simulink model "PlantnMPC"  (R2020b)
settings: Solver=VariableStepAuto  StartTime=0.0  StopTime=100  RelTol=1e-3
undefined symbols (not defined in the file): dU0, magnitude, U0
settings Model: Creator=firda  LastModifiedBy=firda

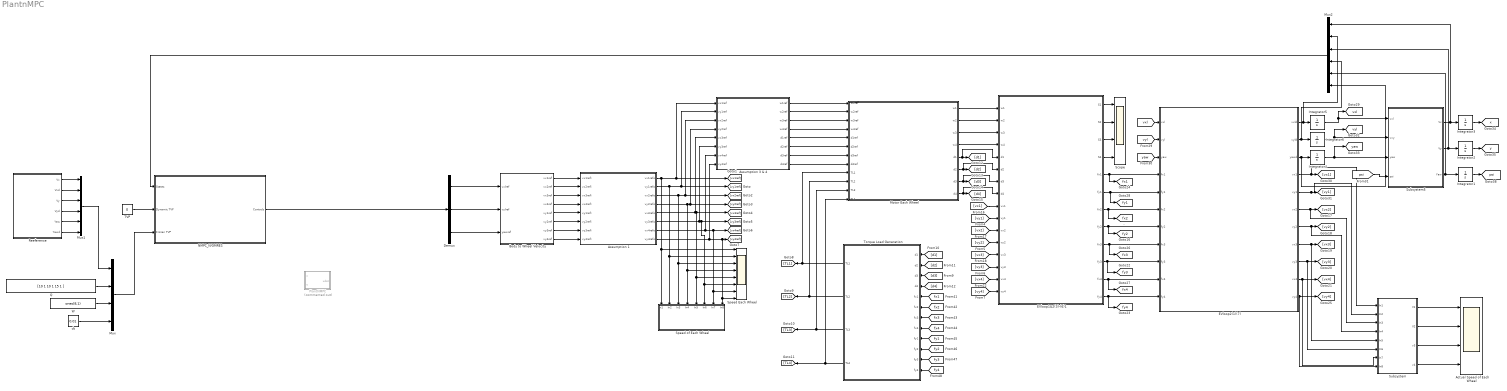
== system PlantnMPC ==
  Actual Speed of Each Wheel : Scope  NumInputPorts=4
  Assumption 1 : Subsystem  mask(Ketentuan ICM){}
      mask help:
      | djref tidak terdefinisi ketika vxjref=vyjref=0
      | vxjref dan vyjref mengambil nilai sebelumnya saat keduanya sama dengan nol
  Assumption 3 & 4 : Subsystem  mask(Persamaan ICM){rej=0.32}
      mask prompts: rej "Jari-jari roda (m)"
      mask help:
      | Asumsi 3 (Zero Slip), bidang roda berhimpit dengan Vj, aj=0,
      | djref=sudut apit (vxjref dan vyjref)
      | Asumsi 4 (Free Rolling), slip longitudinal SLj=0,
      | wjref= norm(vxjref,vyjref)/rej
  Body to Wheel Velocity : Subsystem  mask(Persamaan ICM){ld=0.75, lf=1.42, lr=1.42}
      mask prompts: ld "Jarak pusat masa ke bodi samping (m)"; lf "Jarak pusat masa ke bodi depan (m)"; lr "Jarak pusat masa ke bodi belakang (m)"
      mask help:
      | mengkoordinasikan kecepatan masing-masing roda
      | terhadap kecepatan pusat kendaraan
      | dengan menggunakan konsep ICM
  Demux : Demux  Outputs=3
  EVloop1&2(3)-(6)1 : Subsystem  mask(Vehicle body dinamic){re1=0.32, re2=0.32, re3=0.32, re4=0.32, m=1000, g=9.8, h=0.42, ld=0.75, lf=1.42, lr=1.42, kro=20972, kfo=50539, ksj=0.95}
      mask prompts: re1 "jari-jari roda 1 (m)"; re2 "jari-jari roda 2 (m)"; re3 "jari-jari roda 3 (m)"; re4 "jari-jari roda 4 (m)"; m "massa kendaraan (kg)"; g "percepatan gravitasi (m/s^2)"; h "tinggi pusat massa dari permukaan jalan (m)"; ld "jarak pusat massa ke bodi samping (m)"; lf "jarak pusat massa ke bodi depan (m)"; lr "jarak pusat massa ke bodi belakang (m)"; kro "ketegangan roll belakang"; kfo "ketegangan roll depan"; ksj "faktor atenuasi"
      mask help: Persamaan (3)(4)(5)(6)
  EVloop2(1)(7) : Subsystem  mask(Vehicle bodi dinamic){m=1000, ld=0.75, lf=1.42, lr=1.42, Jz=1950}
      mask prompts: m "massa kendaraan (kg)"; ld "jarak pusat massa ke bodi samping (m)"; lf "jarak pusat massa ke bodi depan (m)"; lr "jarak pusat massa ke bodi belakang (m)"; Jz "the moment of inertia of the vehicle about an axis through its CM"
      mask help: Loop 2 Persamaan 1 & 7
  Integrator{1..4,6} (5 alike) : Integrator
  Integrator5 : Integrator  InitialCondition=1.6
  Motor Each Wheel : Subsystem
      mask Display: image('C:\Users\firda\Desktop\Scenario\4wheels.jpg'); % Use "Edit Image" on toolstrip to change.
  Mux : Mux
  Mux1 : Mux  Inputs=6
  Mux2 : Mux  Inputs=6
  NMPC_N/GMRES : Subsystem
  PlantNMPC : MATLAB Function  Commented=on  TreatAsAtomicUnit=on
  Q : Constant  Value=[10 1 10 1 15 1 ]
  Reeference : Subsystem
      mask Display: image('Reference.jpg'); % Use "Edit Image" on toolstrip to change.
  Scope : Scope  NumInputPorts=4
  Speed Each Wheel : Scope  NumInputPorts=8
  Speed of Each Wheel : Subsystem
  Subsystem : Subsystem
  Subsystem5 : Subsystem
  TVP : Constant  Value=0
  Torque Load Generation : Subsystem  mask(Vehicle body dinamic){jm1=0.36, jm2=0.36, jm3=0.36, jm4=0.36, re1=0.32, re2=0.32, re3=0.32, re4=0.32}
      mask prompts: jm1 "momen inersia roda 1 (kgm^2)"; jm2 "momen inersia roda 2 (kgm^2)"; jm3 "momen inersia roda 3 (kgm^2)"; jm4 "momen inersia roda 4 (kgm^2)"; re1 "jari-jari roda 1 (m)"; re2 "jari-jari roda 2 (m)"; re3 "jari-jari roda 3 (m)"; re4 "jari-jari roda 4 (m)"
      mask help: Persamaan (9)
  W : Constant  Value=ones(8,1)
  dt : Constant  Value=0.01
  tag scope: fx1=global, fx2=global, fx3=global, fx4=global, fy1=global, fy2=global, fy3=global, fy4=global, psi=global, vxl=global, vyl=global, x=global, y=global, yaw=global
  wires:
  Assumption 1/1(vx1refo) -> Assumption 3 & 4/1(vx1ref), [vx1ref], Speed of Each Wheel/1(In1), Speed Each Wheel/1
  Assumption 1/2(vy1refo) -> Assumption 3 & 4/2(vy1ref), [vy1ref], Speed Each Wheel/2, Speed of Each Wheel/2(In2)
  Assumption 1/3(vx2refo) -> Assumption 3 & 4/3(vx2ref), [vx2ref], Speed Each Wheel/3, Speed of Each Wheel/3(In3)
  Assumption 1/4(vy2refo) -> [vy2ref], Assumption 3 & 4/4(vy2ref), Speed of Each Wheel/4(In4), Speed Each Wheel/4
  Assumption 1/5(vx3refo) -> Speed Each Wheel/5, Speed of Each Wheel/5(In5), [vx3ref], Assumption 3 & 4/5(vx3ref)
  Assumption 1/6(vy3refo) -> [vy3ref], Speed Each Wheel/6, Speed of Each Wheel/6(In6), Assumption 3 & 4/6(vy3ref)
  Assumption 1/7(vx4refo) -> [vx4ref], Speed Each Wheel/7, Speed of Each Wheel/7(In7), Assumption 3 & 4/7(vx4ref)
  Assumption 1/8(vy4refo) -> Speed Each Wheel/8, Speed of Each Wheel/8(In8), [vy4ref], Assumption 3 & 4/8(vy4ref)
  Assumption 3 & 4/1(w1ref) -> Motor Each Wheel/1(w1ref)
  Assumption 3 & 4/2(w2ref) -> Motor Each Wheel/2(w2ref)
  Assumption 3 & 4/3(w3ref) -> Motor Each Wheel/3(w3ref)
  Assumption 3 & 4/4(w4ref) -> Motor Each Wheel/4(w4ref)
  Assumption 3 & 4/5(d1ref) -> Motor Each Wheel/5(d1ref)
  Assumption 3 & 4/6(d2ref) -> Motor Each Wheel/6(d2ref)
  Assumption 3 & 4/7(d3ref) -> Motor Each Wheel/7(d3ref)
  Assumption 3 & 4/8(d4ref) -> Motor Each Wheel/8(d4ref)
  Torque Load Generation/3(TL3) -> Motor Each Wheel/11(TL3), [TL3]
  Torque Load Generation/4(TL4) -> Motor Each Wheel/12(TL4), [TL4]
  Torque Load Generation/1(TL1) -> Motor Each Wheel/9(TL1), [TL1]
  [d1] -> Torque Load Generation/1(d1)
  [d2] -> Torque Load Generation/2(d2)
  [d3] -> Torque Load Generation/3(d3)
  [d4] -> Torque Load Generation/4(d4)
  [fx1] -> Torque Load Generation/5(fx1)
  [fx2] -> Torque Load Generation/6(fx2)
  [fx3] -> Torque Load Generation/7(fx3)
  [fx4] -> Torque Load Generation/8(fx4)
  [fy1] -> Torque Load Generation/9(fy1)
  [fy2] -> Torque Load Generation/10(fy2)
  [fy3] -> Torque Load Generation/11(fy3)
  [fy4] -> Torque Load Generation/12(fy4)
  Torque Load Generation/2(TL2) -> [TL2], Motor Each Wheel/10(TL2)
  Motor Each Wheel/1(w1) -> EVloop1&2(3)-(6)1/1(w1)
  Motor Each Wheel/2(w2) -> EVloop1&2(3)-(6)1/2(w2)
  Motor Each Wheel/3(w3) -> EVloop1&2(3)-(6)1/3(w3)
  Motor Each Wheel/4(w4) -> EVloop1&2(3)-(6)1/4(w4)
  Motor Each Wheel/6(d2) -> EVloop1&2(3)-(6)1/6(d2), [d2]
  Motor Each Wheel/7(d3) -> EVloop1&2(3)-(6)1/7(d3), [d3]
  Motor Each Wheel/8(d4) -> EVloop1&2(3)-(6)1/8(d4), [d4]
  Motor Each Wheel/5(d1) -> EVloop1&2(3)-(6)1/5(d1), [d1]
  [vx1] -> EVloop1&2(3)-(6)1/9(vx1)
  [vy1] -> EVloop1&2(3)-(6)1/10(vy1)
  [vx2] -> EVloop1&2(3)-(6)1/11(vx2)
  [vy4] -> EVloop1&2(3)-(6)1/16(vy4)
  [vx4] -> EVloop1&2(3)-(6)1/15(vx4)
  [vy3] -> EVloop1&2(3)-(6)1/14(vy3)
  [vx3] -> EVloop1&2(3)-(6)1/13(vx3)
  [vy2] -> EVloop1&2(3)-(6)1/12(vy2)
  EVloop1&2(3)-(6)1/1(S1) -> Scope/1
  EVloop1&2(3)-(6)1/2(S2) -> Scope/2
  EVloop1&2(3)-(6)1/3(S3) -> Scope/3
  EVloop1&2(3)-(6)1/4(S4) -> Scope/4
  EVloop1&2(3)-(6)1/5(fx1) -> [fx1], EVloop2(1)(7)/4(fx1)
  EVloop1&2(3)-(6)1/6(fy1) -> [fy1], EVloop2(1)(7)/5(fy1)
  EVloop1&2(3)-(6)1/7(fx2) -> [fx2], EVloop2(1)(7)/6(fx2)
  EVloop1&2(3)-(6)1/8(fy2) -> [fy2], EVloop2(1)(7)/7(fy2)
  EVloop1&2(3)-(6)1/9(fx3) -> [fx3], EVloop2(1)(7)/8(fx3)
  EVloop1&2(3)-(6)1/10(fy3) -> [fy3], EVloop2(1)(7)/9(fy3)
  EVloop1&2(3)-(6)1/11(fx4) -> [fx4], EVloop2(1)(7)/10(fx4)
  EVloop1&2(3)-(6)1/12(fy4) -> [fy4], EVloop2(1)(7)/11(fy4)
  [vxl] -> EVloop2(1)(7)/1(vxl)
  [vyl] -> EVloop2(1)(7)/2(vyl)
  [yaw] -> EVloop2(1)(7)/3(yaw)
  Integrator4/1 -> Subsystem5/3(yaw), [yaw]
  Integrator6/1 -> Subsystem5/2(vxy), [vyl]
  Integrator5/1 -> Subsystem5/1(vxl), [vxl]
  EVloop2(1)(7)/1(vxld) -> Mux2/2, Integrator5/1
  EVloop2(1)(7)/2(vyld) -> Mux2/4, Integrator6/1
  EVloop2(1)(7)/3(yawd) -> Mux2/6, Integrator4/1
  [psi] -> Subsystem5/4(psi)
  Integrator2/1 -> [y]
  Subsystem5/1(Vx) -> Mux2/1, Integrator3/1
  Integrator3/1 -> [x]
  Integrator1/1 -> [psi]
  Subsystem5/2(Vy) -> Mux2/3, Integrator2/1
  Subsystem5/3(Yaw) -> Integrator1/1, Mux2/5
  EVloop2(1)(7)/4(vx1) -> Subsystem/1(In1), [vx1]
  EVloop2(1)(7)/5(vy1) -> Subsystem/2(In2), [vy1]
  EVloop2(1)(7)/6(vx2) -> Subsystem/3(In3), [vx2]
  EVloop2(1)(7)/7(vy2) -> Subsystem/4(In4), [vy2]
  EVloop2(1)(7)/8(vx3) -> Subsystem/5(In5), [vx3]
  EVloop2(1)(7)/9(vy3) -> Subsystem/6(In6), [vy3]
  EVloop2(1)(7)/10(vx4) -> Subsystem/7(In7), [vx4]
  EVloop2(1)(7)/11(vy4) -> Subsystem/8(In8), [vy4]
  Subsystem/1(V1) -> Actual Speed of Each Wheel/1
  Subsystem/2(V2) -> Actual Speed of Each Wheel/2
  Subsystem/3(v3) -> Actual Speed of Each Wheel/3
  Subsystem/4(v4) -> Actual Speed of Each Wheel/4
  Body to Wheel Velocity/8(vy4ref) -> Assumption 1/8(vy4refi)
  Body to Wheel Velocity/7(vy3ref) -> Assumption 1/7(vy3refi)
  Body to Wheel Velocity/6(vy2ref) -> Assumption 1/6(vy2refi)
  Body to Wheel Velocity/5(vy1ref) -> Assumption 1/5(vy1refi)
  Body to Wheel Velocity/4(vx4ref) -> Assumption 1/4(vx4refi)
  Body to Wheel Velocity/3(vx3ref) -> Assumption 1/3(vx3refi)
  Body to Wheel Velocity/2(vx2ref) -> Assumption 1/2(vx2refi)
  Body to Wheel Velocity/1(vx1ref) -> Assumption 1/1(vx1refi)
  Demux/1 -> Body to Wheel Velocity/1(vxlref)
  Demux/2 -> Body to Wheel Velocity/2(vylref)
  Demux/3 -> Body to Wheel Velocity/3(yawref)
  Q/1 -> Mux/2
  dt/1 -> Mux/4
  W/1 -> Mux/3
  Mux/1 -> NMPC_N/GMRES/3(Frozen TVP)
  Mux1/1 -> Mux/1
  Reeference/1(Vx) -> Mux1/1
  Reeference/2(Vxd) -> Mux1/2
  Reeference/3(Vy) -> Mux1/3
  Reeference/4(Vyd) -> Mux1/4
  Reeference/5(Yaw) -> Mux1/5
  Reeference/6(Yawd) -> Mux1/6
  TVP/1 -> NMPC_N/GMRES/2(Dynamic TVP)
  NMPC_N/GMRES/1(Controls) -> Demux/1
  Mux2/1 -> NMPC_N/GMRES/1(States)

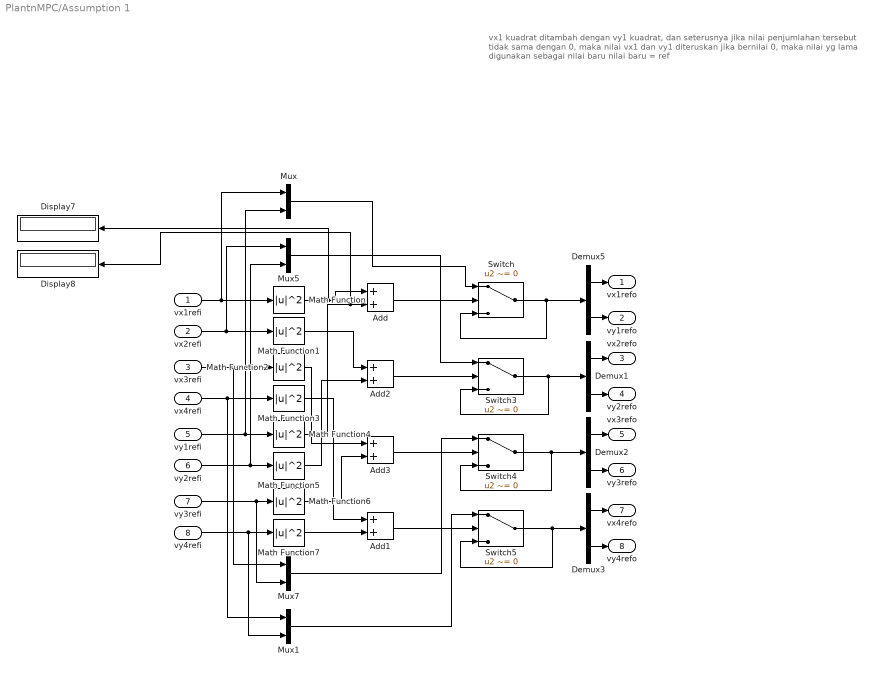
== system PlantnMPC/Assumption 1 ==
  note: vx1 kuadrat ditambah dengan vy1 kuadrat, dan seterusnya
      | jika nilai penjumlahan tersebut tidak sama dengan 0, maka nilai vx1 dan vy1 diteruskan
      | jika bernilai 0, maka nilai yg lama digunakan sebagai nilai baru
      | nilai baru = ref
  vx1refi : Inport
  vx2refi : Inport  Port=2
  vx3refi : Inport  Port=3
  vx4refi : Inport  Port=4
  vy1refi : Inport  Port=5
  vy2refi : Inport  Port=6
  vy3refi : Inport  Port=7
  vy4refi : Inport  Port=8
  Add{,1..3} (4 alike) : Sum
  Demux{1..3,5} (4 alike) : Demux  Outputs=2
  Display7 : Display
  Display8 : Display
  Math Function{,1..7} (8 alike) : Math  Operator=magnitude^2  SignedPower=on  SaturateOnIntegerOverflow=on
  Mux{,1,5,7} (4 alike) : Mux  Inputs=2
  Switch{,3..5} (4 alike) : Switch  Criteria=u2 ~= 0
  vx1refo : Outport
  vy1refo : Outport  Port=2
  vx2refo : Outport  Port=3
  vy2refo : Outport  Port=4
  vx3refo : Outport  Port=5
  vy3refo : Outport  Port=6
  vx4refo : Outport  Port=7
  vy4refo : Outport  Port=8
  wires:
  Add2/1 -> Switch3/2
  Switch3/1 -> Switch3/3, Demux1/1
  Math Function3/1 -> Add1/1
  Demux3/2 -> vy4refo/1
  Demux5/1 -> vx1refo/1
  Demux2/1 -> vx3refo/1
  Demux3/1 -> vx4refo/1
  Math Function5/1 -> Add2/2
  vx3refi/1 -> Mux7/1, Math Function2/1
  Switch4/1 -> Switch4/3, Demux2/1
  vx2refi/1 -> Math Function1/1, Mux5/1
  Math Function6/1 -> Add3/2
  vy4refi/1 -> Mux1/2, Math Function7/1
  Math Function/1 -> Display7/1, Add/1
  Mux5/1 -> Switch3/1
  Add/1 -> Switch/2
  Mux7/1 -> Switch4/1
  Add3/1 -> Switch4/2
  Switch5/1 -> Switch5/3, Demux3/1
  Math Function2/1 -> Add3/1
  vx4refi/1 -> Mux1/1, Math Function3/1
  vy3refi/1 -> Mux7/2, Math Function6/1
  vy2refi/1 -> Mux5/2, Math Function5/1
  Math Function1/1 -> Add2/1
  Switch/1 -> Switch/3, Demux5/1
  vx1refi/1 -> Mux/1, Math Function/1
  Math Function4/1 -> Display8/1, Add/2
  vy1refi/1 -> Mux/2, Math Function4/1
  Mux/1 -> Switch/1
  Math Function7/1 -> Add1/2
  Add1/1 -> Switch5/2
  Demux1/1 -> vx2refo/1
  ? -> ?
  Mux1/1 -> Switch5/1
  Demux5/2 -> vy1refo/1
  Demux2/2 -> vy3refo/1
  Demux1/2 -> vy2refo/1

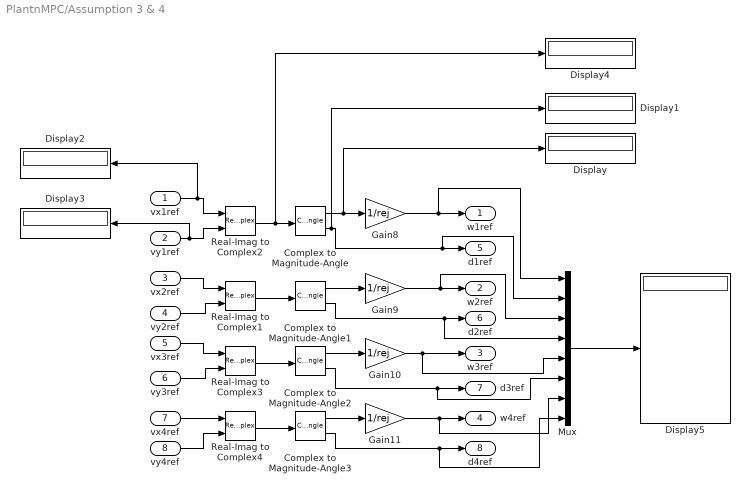
== system PlantnMPC/Assumption 3 & 4 ==
  vx1ref : Inport
  vy1ref : Inport  Port=2
  vx2ref : Inport  Port=3
  vy2ref : Inport  Port=4
  vx3ref : Inport  Port=5
  vy3ref : Inport  Port=6
  vx4ref : Inport  Port=7
  vy4ref : Inport  Port=8
  Complex to Magnitude-Angle{,1..3} (4 alike) : ComplexToMagnitudeAngle
  Display{,1..5} (6 alike) : Display
  Gain{8..11} (4 alike) : Gain  Gain=1/rej
  Mux : Mux  Inputs=8
  Real-Imag to Complex{1..4} (4 alike) : RealImagToComplex
  w1ref : Outport
  w2ref : Outport  Port=2
  w3ref : Outport  Port=3
  w4ref : Outport  Port=4
  d1ref : Outport  Port=5
  d2ref : Outport  Port=6
  d3ref : Outport  Port=7
  d4ref : Outport  Port=8
  wires:
  vx2ref/1 -> Real-Imag to Complex1/1
  vy1ref/1 -> Real-Imag to Complex2/2, Display3/1
  Gain8/1 -> Mux/1, w1ref/1
  Complex to Magnitude-Angle/2 -> Display1/1, Mux/2, d1ref/1
  Gain9/1 -> Mux/3, w2ref/1
  vy2ref/1 -> Real-Imag to Complex1/2
  Complex to Magnitude-Angle2/2 -> Mux/6, d3ref/1
  vx3ref/1 -> Real-Imag to Complex3/1
  vy4ref/1 -> Real-Imag to Complex4/2
  Complex to Magnitude-Angle3/1 -> Gain11/1
  Complex to Magnitude-Angle3/2 -> Mux/8, d4ref/1
  Real-Imag to Complex1/1 -> Complex to Magnitude-Angle1/1
  Complex to Magnitude-Angle1/2 -> Mux/4, d2ref/1
  vy3ref/1 -> Real-Imag to Complex3/2
  Complex to Magnitude-Angle/1 -> Display/1, Gain8/1
  Gain11/1 -> Mux/7, w4ref/1
  vx1ref/1 -> Display2/1, Real-Imag to Complex2/1
  vx4ref/1 -> Real-Imag to Complex4/1
  Real-Imag to Complex2/1 -> Display4/1, Complex to Magnitude-Angle/1
  Complex to Magnitude-Angle1/1 -> Gain9/1
  Real-Imag to Complex3/1 -> Complex to Magnitude-Angle2/1
  Complex to Magnitude-Angle2/1 -> Gain10/1
  Real-Imag to Complex4/1 -> Complex to Magnitude-Angle3/1
  Gain10/1 -> w3ref/1, Mux/5
  Mux/1 -> Display5/1

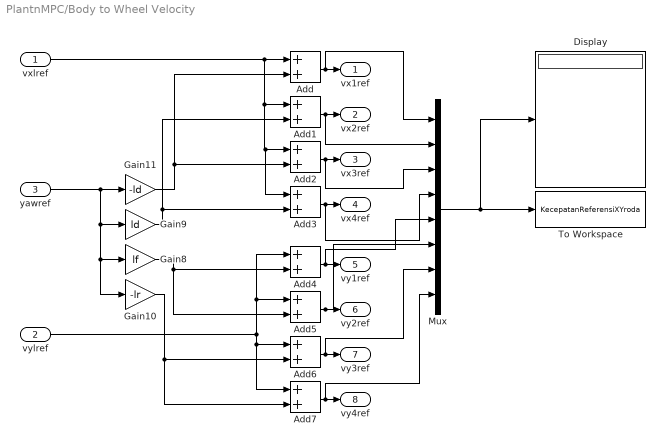
== system PlantnMPC/Body to Wheel Velocity ==
  vxlref : Inport
  vylref : Inport  Port=2
  yawref : Inport  Port=3
  Add{,1..7} (8 alike) : Sum
  Display : Display
  Gain10 : Gain  Gain=-lr
  Gain11 : Gain  Gain=-ld
  Gain8 : Gain  Gain=lf
  Gain9 : Gain  Gain=ld
  Mux : Mux  Inputs=8
  To Workspace : ToWorkspace  VariableName=KecepatanReferensiXYroda  SaveFormat=Structure With Time  SampleTime=0.01
  vx1ref : Outport
  vx2ref : Outport  Port=2
  vx3ref : Outport  Port=3
  vx4ref : Outport  Port=4
  vy1ref : Outport  Port=5
  vy2ref : Outport  Port=6
  vy3ref : Outport  Port=7
  vy4ref : Outport  Port=8
  wires:
  Gain10/1 -> Add7/2, Add6/2
  Add1/1 -> Mux/2, vx2ref/1
  Gain8/1 -> Add4/2, Add5/2
  yawref/1 -> Gain9/1, Gain8/1, Gain10/1, Gain11/1
  vylref/1 -> Add7/1, Add6/1, Add5/1, Add4/1
  vxlref/1 -> Add3/1, Add2/1, Add1/1, Add/1
  Gain9/1 -> Add1/2, Add3/2
  Gain11/1 -> Add2/2, Add/2
  Add3/1 -> Mux/4, vx4ref/1
  Add/1 -> Mux/1, vx1ref/1
  Add5/1 -> Mux/6, vy2ref/1
  Add2/1 -> Mux/3, vx3ref/1
  Add4/1 -> Mux/5, vy1ref/1
  Add6/1 -> Mux/7, vy3ref/1
  Add7/1 -> Mux/8, vy4ref/1
  Mux/1 -> Display/1, To Workspace/1

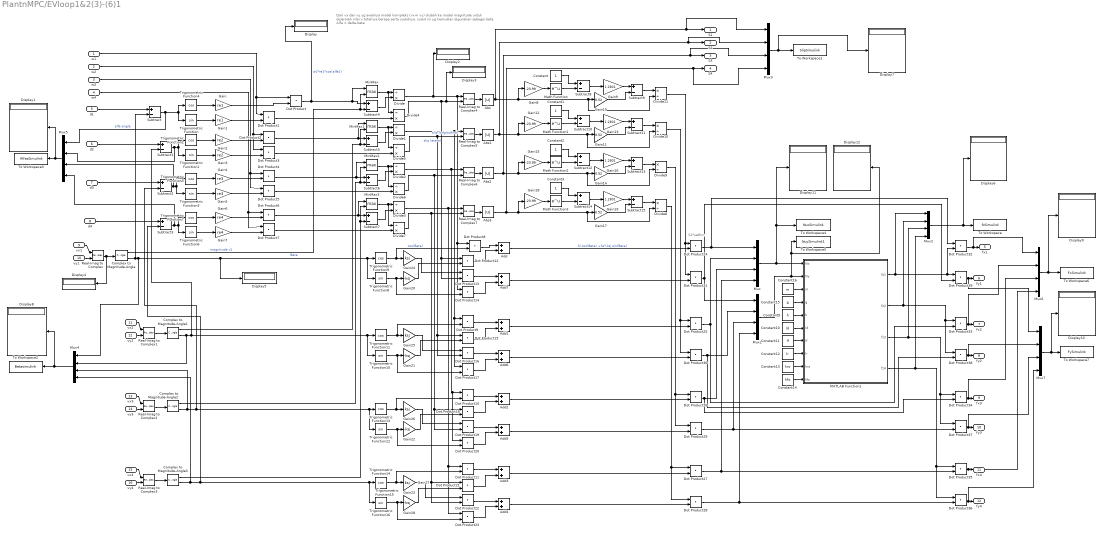
== system PlantnMPC/EVloop1&2(3)-(6)1 ==
  note: S1*satfcn
  note: Dari vx dan vy yg awalnya model kompleks (vx+i vy) diubah ke model magnitude untuk diperoleh nilai v totalnya berapa serta sudutnya. sudut ini yg kemudian digunakan sebagai beta.
      | Alfa = delta-beta
  w1 : Inport
  w2 : Inport  Port=2
  w3 : Inport  Port=3
  w4 : Inport  Port=4
  d1 : Inport  Port=5
  d2 : Inport  Port=6
  d3 : Inport  Port=7
  d4 : Inport  Port=8
  vx1 : Inport  Port=9
  vy1 : Inport  Port=10
  vx2 : Inport  Port=11
  vy2 : Inport  Port=12
  vx3 : Inport  Port=13
  vy3 : Inport  Port=14
  vx4 : Inport  Port=15
  vy4 : Inport  Port=16
  Abs{,1..3} (4 alike) : Abs
  Add{,1..7} (8 alike) : Sum
  Complex to Magnitude-Angle{,1..3} (4 alike) : ComplexToMagnitudeAngle
  Constant{,1..3} (4 alike) : Constant
  Constant10 : Constant  Value=ld
  Constant11 : Constant  Value=lf
  Constant12 : Constant  Value=lr
  Constant13 : Constant  Value=kro
  Constant14 : Constant  Value=kfo
  Constant15 : Constant  Value=g
  Constant16 : Constant  Value=m
  Constant9 : Constant  Value=h
  Display{,1..12} (13 alike) : Display
  Divide{,1..7} (8 alike) : Product  Inputs=/*
  Divide{8..11} (4 alike) : Product  Inputs=*/
  Dot Product{,1..39} (40 alike) : DotProduct  InputSameDT=on  OutDataTypeStr=Inherit: Inherit via internal rule
  Gain : Gain  Gain=re1
  Gain1 : Gain  Gain=re1
  Gain{10..11,14,17} (4 alike) : Gain  Gain=0.52
  Gain{8,12,15,18} (4 alike) : Gain  Gain=-23.99
  Gain{9,13,16,19} (4 alike) : Gain  Gain=1.2801
  Gain2 : Gain  Gain=re2
  Gain{20..23,28} (5 alike) : Gain  Gain=-ksj
  Gain{24..27} (4 alike) : Gain  Gain=ksj
  Gain3 : Gain  Gain=re2
  Gain4 : Gain  Gain=re3
  Gain5 : Gain  Gain=re3
  Gain6 : Gain  Gain=re4
  Gain7 : Gain  Gain=re4
  MATLAB Function1 : MATLAB Function  TreatAsAtomicUnit=on
  Math Function{,1..3} (4 alike) : Math  SignedPower=on  SaturateOnIntegerOverflow=on
  MinMax{,1..3} (4 alike) : MinMax  Function=max  Inputs=2
  Mux{,1..7} (8 alike) : Mux
  Real-Imag to Complex{,1..7} (8 alike) : RealImagToComplex
  Subtract{,1..15} (16 alike) : Sum  Inputs=+-
  To Workspace : ToWorkspace  VariableName=fzSimulink  SaveFormat=Structure With Time  SampleTime=0.01
      settings: Save2DSignal=2-D array (concatenate along first dimension)
  To Workspace1 : ToWorkspace  VariableName=SlipSimulink  SaveFormat=Structure With Time  SampleTime=0.01
  To Workspace2 : ToWorkspace  VariableName=Betasimulink  SaveFormat=Structure With Time  SampleTime=0.01
  To Workspace3 : ToWorkspace  VariableName=AlfasSimulink  SaveFormat=Structure With Time  SampleTime=0.01
  To Workspace4 : ToWorkspace  VariableName=NuxSimulink  SaveFormat=Structure With Time  SampleTime=0.01
  To Workspace5 : ToWorkspace  VariableName=NuySimulink1  SaveFormat=Structure With Time  SampleTime=0.01
  To Workspace6 : ToWorkspace  VariableName=FxSimulink  SaveFormat=Structure With Time  SampleTime=0.01
  To Workspace7 : ToWorkspace  VariableName=FySimulink  SaveFormat=Structure With Time  SampleTime=0.01
  Trigonometric Function{,1,3,6,8,10,12,14,16} (9 alike) : Trigonometry
  Trigonometric Function{2,4..5,7,9,11,13,15} (8 alike) : Trigonometry  Operator=cos
  S1 : Outport
  S2 : Outport  Port=2
  S3 : Outport  Port=3
  S4 : Outport  Port=4
  fx1 : Outport  Port=5
  fy1 : Outport  Port=6
  fx2 : Outport  Port=7
  fy2 : Outport  Port=8
  fx3 : Outport  Port=9
  fy3 : Outport  Port=10
  fx4 : Outport  Port=11
  fy4 : Outport  Port=12
  wires:
  Dot Product33/1 -> Mux6/2, fx2/1
  Dot Product35/1 -> Mux6/4, fx4/1
  Dot Product28/1 -> Dot Product36/2, Mux1/4
  Dot Product36/1 -> Mux7/4, fy4/1
  Dot Product34/1 -> Mux6/3, fx3/1
  Dot Product39/1 -> Mux7/1, fy1/1
  Dot Product37/1 -> Mux7/3, fy3/1
  Dot Product38/1 -> Mux7/2, fy2/1
  Dot Product32/1 -> Mux6/1, fx1/1
  vx1/1 -> Real-Imag to Complex/1
  vy1/1 -> Real-Imag to Complex/2
  vx3/1 -> Real-Imag to Complex2/1
  vy3/1 -> Real-Imag to Complex2/2
  vx4/1 -> Real-Imag to Complex3/1
  vx2/1 -> Real-Imag to Complex1/1
  vy4/1 -> Real-Imag to Complex3/2
  vy2/1 -> Real-Imag to Complex1/2
  Constant15/1 -> MATLAB Function1/4(g)
  Dot Product31/1 -> Dot Product39/2, Mux1/1
  Dot Product29/1 -> Dot Product37/2, Mux1/3
  Dot Product30/1 -> Dot Product38/2, Mux1/2
  Constant16/1 -> MATLAB Function1/3(m)
  MATLAB Function1/1(fz1) -> Mux2/1, Dot Product32/2, Dot Product39/1
  MATLAB Function1/3(fz3) -> Mux2/3, Dot Product34/1, Dot Product37/1
  Constant14/1 -> MATLAB Function1/10(kfo)
  Constant13/1 -> MATLAB Function1/9(kro)
  Real-Imag to Complex2/1 -> Complex to Magnitude-Angle2/1
  Real-Imag to Complex3/1 -> Complex to Magnitude-Angle3/1
  Complex to Magnitude-Angle/2 -> Mux4/1, Display5/1, Trigonometric Function8/1, Trigonometric Function9/1, Subtract/2  "Beta"
  Complex to Magnitude-Angle1/2 -> Mux4/2, Trigonometric Function10/1, Trigonometric Function11/1, Subtract1/2
  Real-Imag to Complex/1 -> Display4/1, Complex to Magnitude-Angle/1
  Real-Imag to Complex1/1 -> Complex to Magnitude-Angle1/1
  Trigonometric Function1/1 -> Gain3/1
  w1/1 -> Dot Product1/1, Dot Product/1
  Trigonometric Function5/1 -> Gain4/1
  d4/1 -> Subtract3/1
  Subtract/1 -> Mux5/1, Trigonometric Function/1, Trigonometric Function4/1  "alfa angle"
  Gain4/1 -> Dot Product4/2
  w2/1 -> Dot Product2/1, Dot Product3/1
  w4/1 -> Dot Product6/1, Dot Product7/1
  Subtract2/1 -> Mux5/3, Trigonometric Function3/1, Trigonometric Function5/1
  d3/1 -> Subtract2/1
  Gain5/1 -> Dot Product5/2
  Gain/1 -> Dot Product/2
  Dot Product2/1 -> MinMax1/1, Subtract5/1
  Gain1/1 -> Dot Product1/2
  d1/1 -> Subtract/1
  Gain3/1 -> Dot Product3/2
  Gain7/1 -> Dot Product7/2
  Trigonometric Function6/1 -> Gain7/1
  Dot Product/1 -> Display/1, Subtract4/1, MinMax/1  "w1*re1*cos(alfa1)"
  Complex to Magnitude-Angle3/2 -> Mux4/4, Subtract3/2, Trigonometric Function16/1, Trigonometric Function14/1, Trigonometric Function15/1
  Trigonometric Function4/1 -> Gain/1
  Complex to Magnitude-Angle2/2 -> Mux4/3, Trigonometric Function12/1, Trigonometric Function13/1, Subtract2/2
  Subtract1/1 -> Mux5/2, Trigonometric Function2/1, Trigonometric Function1/1
  Trigonometric Function2/1 -> Gain2/1
  Trigonometric Function3/1 -> Gain5/1
  Gain6/1 -> Dot Product6/2
  Trigonometric Function/1 -> Gain1/1
  Gain2/1 -> Dot Product2/2
  w3/1 -> Dot Product4/1, Dot Product5/1
  Trigonometric Function7/1 -> Gain6/1
  d2/1 -> Subtract1/1
  Subtract3/1 -> Mux5/4, Trigonometric Function6/1, Trigonometric Function7/1
  Complex to Magnitude-Angle/1 -> MinMax/2, Subtract4/2  "magnitude v1"
  Real-Imag to Complex5/1 -> Abs1/1
  Divide3/1 -> Dot Product23/1, Dot Product11/1, Real-Imag to Complex7/1
  Dot Product5/1 -> Divide6/2
  Divide/1 -> Display2/1, Dot Product14/1, Dot Product8/1, Real-Imag to Complex4/1  "slip longitudinal"
  Real-Imag to Complex6/1 -> Abs2/1
  MinMax3/1 -> Divide7/1, Divide3/1
  Divide7/1 -> Dot Product22/2, Dot Product21/1, Real-Imag to Complex7/2
  MinMax1/1 -> Divide5/1, Divide1/1
  Dot Product3/1 -> Divide5/2
  Dot Product7/1 -> Divide7/2
  Subtract5/1 -> Divide1/2
  Divide6/1 -> Dot Product19/2, Dot Product18/1, Real-Imag to Complex6/2
  Real-Imag to Complex7/1 -> Abs3/1
  Complex to Magnitude-Angle3/1 -> MinMax3/2, Subtract7/2
  Dot Product4/1 -> MinMax2/1, Subtract6/1
  Dot Product6/1 -> MinMax3/1, Subtract7/1
  Real-Imag to Complex4/1 -> Abs/1
  Gain8/1 -> Math Function/1
  Subtract6/1 -> Divide2/2
  Math Function/1 -> Subtract8/2
  Divide4/1 -> Dot Product13/2, Dot Product12/1, Display3/1, Real-Imag to Complex4/2  "slip lateral"
  Complex to Magnitude-Angle2/1 -> MinMax2/2, Subtract6/2
  Dot Product1/1 -> Divide4/2
  Subtract4/1 -> Divide/2
  Complex to Magnitude-Angle1/1 -> MinMax1/2, Subtract5/2
  MinMax/1 -> Divide4/1, Divide/1
  Subtract7/1 -> Divide3/2
  Divide5/1 -> Dot Product15/1, Dot Product16/2, Real-Imag to Complex5/2
  Divide2/1 -> Dot Product20/1, Dot Product10/1, Real-Imag to Complex6/1
  MinMax2/1 -> Divide6/1, Divide2/1
  Divide1/1 -> Dot Product9/1, Dot Product17/1, Real-Imag to Complex5/1
  Gain9/1 -> Subtract9/1
  Gain12/1 -> Math Function1/1
  Trigonometric Function8/1 -> Dot Product14/2, Gain20/1
  Trigonometric Function10/1 -> Dot Product17/2, Gain21/1
  Gain10/1 -> Subtract9/2
  Subtract8/1 -> Gain9/1
  Trigonometric Function14/1 -> Gain23/1
  Subtract14/1 -> Gain19/1
  Abs3/1 -> Mux3/4, S4/1, Gain18/1, Gain17/1, Divide8/2
  Abs2/1 -> Mux3/3, S3/1, Gain15/1, Divide9/2, Gain14/1
  Subtract13/1 -> Divide9/1
  Subtract10/1 -> Gain13/1
  Gain18/1 -> Math Function3/1
  Subtract15/1 -> Divide8/1
  Constant2/1 -> Subtract12/1
  Constant1/1 -> Subtract10/1
  Constant3/1 -> Subtract14/1
  Trigonometric Function12/1 -> Dot Product20/2, Gain22/1
  Abs1/1 -> Mux3/2, S2/1, Gain12/1, Divide10/2, Gain11/1
  Trigonometric Function9/1 -> Dot Product8/2, Gain24/1  "cos(Beta)"
  Gain16/1 -> Subtract13/1
  Gain17/1 -> Subtract15/2
  Constant/1 -> Subtract8/1
  Math Function1/1 -> Subtract10/2
  Gain13/1 -> Subtract11/1
  Math Function2/1 -> Subtract12/2
  Subtract12/1 -> Gain16/1
  Gain15/1 -> Math Function2/1
  Gain14/1 -> Subtract13/2
  Math Function3/1 -> Subtract14/2
  Gain19/1 -> Subtract15/1
  Gain11/1 -> Subtract11/2
  Divide9/1 -> Dot Product26/1, Dot Product29/1
  Dot Product11/1 -> Add3/1
  Trigonometric Function13/1 -> Dot Product10/2, Gain26/1
  Add3/1 -> Dot Product27/2
  Dot Product10/1 -> Add2/1
  Add2/1 -> Dot Product26/2
  Dot Product21/1 -> Add3/2
  Divide8/1 -> Dot Product28/1, Dot Product27/1
  Trigonometric Function16/1 -> Dot Product23/2, Gain28/1
  Gain24/1 -> Dot Product13/1
  Dot Product9/1 -> Add1/1
  Gain25/1 -> Dot Product16/1
  Gain26/1 -> Dot Product19/1
  Add4/1 -> Dot Product28/2
  Divide11/1 -> Dot Product31/1, Dot Product24/1
  Dot Product18/1 -> Add2/2
  Add/1 -> Dot Product24/2  "Sl cos(Beta) +Ss*-ksj sin(Beta)"
  Gain20/1 -> Dot Product12/2
  Dot Product8/1 -> Add/1
  Gain21/1 -> Dot Product15/2
  Gain22/1 -> Dot Product18/2
  Dot Product15/1 -> Add1/2
  Divide10/1 -> Dot Product30/1, Dot Product25/1
  Abs/1 -> Mux3/1, S1/1, Gain8/1, Divide11/2, Gain10/1
  Trigonometric Function11/1 -> Dot Product9/2, Gain25/1
  Gain28/1 -> Dot Product21/2
  Trigonometric Function15/1 -> Dot Product11/2, Gain27/1
  Subtract9/1 -> Divide11/1
  Add1/1 -> Dot Product25/2
  Dot Product12/1 -> Add/2
  Subtract11/1 -> Divide10/1
  Add7/1 -> Dot Product31/2
  Dot Product22/1 -> Add4/1
  Dot Product16/1 -> Add6/1
  Add5/1 -> Dot Product29/2
  Dot Product17/1 -> Add6/2
  Dot Product13/1 -> Add7/1
  Dot Product19/1 -> Add5/1
  Dot Product14/1 -> Add7/2
  Add6/1 -> Dot Product30/2
  Dot Product23/1 -> Add4/2
  Dot Product20/1 -> Add5/2
  Dot Product27/1 -> Dot Product35/2, Mux/4
  Constant11/1 -> MATLAB Function1/7(lf)
  Dot Product25/1 -> Dot Product33/2, Mux/2
  Constant9/1 -> MATLAB Function1/5(h)
  Dot Product24/1 -> Dot Product32/1, Mux/1
  Constant10/1 -> MATLAB Function1/6(ld)
  Mux1/1 -> To Workspace5/1, Display12/1, MATLAB Function1/2(Ny)
  Constant12/1 -> MATLAB Function1/8(lr)
  MATLAB Function1/4(fz4) -> Mux2/4, Dot Product36/1, Dot Product35/1
  MATLAB Function1/2(fz2) -> Mux2/2, Dot Product33/1, Dot Product38/1
  Dot Product26/1 -> Dot Product34/2, Mux/3
  Mux/1 -> Display11/1, To Workspace4/1, MATLAB Function1/1(Nx)
  Mux2/1 -> Display6/1, To Workspace/1
  Mux5/1 -> Display1/1, To Workspace3/1
  Mux3/1 -> Display7/1, To Workspace1/1
  Mux6/1 -> Display9/1, To Workspace6/1
  Mux7/1 -> Display10/1, To Workspace7/1
  Mux4/1 -> Display8/1, To Workspace2/1
  Gain27/1 -> Dot Product22/1

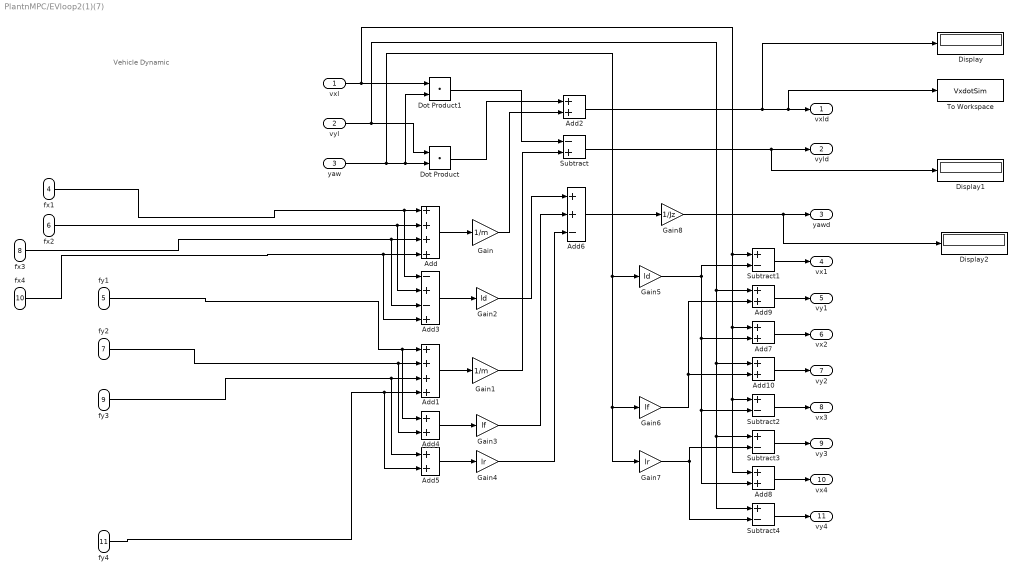
== system PlantnMPC/EVloop2(1)(7) ==
  note: Vehicle Dynamic
  vxl : Inport
  vyl : Inport  Port=2
  yaw : Inport  Port=3
  fx1 : Inport  Port=4
  fy1 : Inport  Port=5
  fx2 : Inport  Port=6
  fy2 : Inport  Port=7
  fx3 : Inport  Port=8
  fy3 : Inport  Port=9
  fx4 : Inport  Port=10
  fy4 : Inport  Port=11
  Add : Sum  Inputs=++++
  Add1 : Sum  Inputs=++++
  Add{2,4..5,7..10} (7 alike) : Sum
  Add3 : Sum  Inputs=-+-+
  Add6 : Sum  Inputs=++-
  Display : Display
  Display1 : Display
  Display2 : Display
  Dot Product : DotProduct  InputSameDT=on  OutDataTypeStr=Inherit: Inherit via internal rule
  Dot Product1 : DotProduct  InputSameDT=on  OutDataTypeStr=Inherit: Inherit via internal rule
  Gain : Gain  Gain=1/m
  Gain1 : Gain  Gain=1/m
  Gain2 : Gain  Gain=ld
  Gain3 : Gain  Gain=lf
  Gain4 : Gain  Gain=lr
  Gain5 : Gain  Gain=ld
  Gain6 : Gain  Gain=lf
  Gain7 : Gain  Gain=lr
  Gain8 : Gain  Gain=1/Jz
  Subtract : Sum  Inputs=-+
  Subtract{1..4} (4 alike) : Sum  Inputs=+-
  To Workspace : ToWorkspace  VariableName=VxdotSim  SaveFormat=Structure With Time  SampleTime=0.01
  vxld : Outport
  vyld : Outport  Port=2
  yawd : Outport  Port=3
  vx1 : Outport  Port=4
  vy1 : Outport  Port=5
  vx2 : Outport  Port=6
  vy2 : Outport  Port=7
  vx3 : Outport  Port=8
  vy3 : Outport  Port=9
  vx4 : Outport  Port=10
  vy4 : Outport  Port=11
  wires:
  Subtract3/1 -> vy3/1
  Add3/1 -> Gain2/1
  Add1/1 -> Gain1/1
  vxl/1 -> Add7/1, Subtract2/1, Add8/1, Subtract1/1, Dot Product1/1
  yaw/1 -> Gain7/1, Gain6/1, Gain5/1, Dot Product1/2, Dot Product/2
  Add8/1 -> vx4/1
  Add/1 -> Gain/1
  Gain6/1 -> Add10/2, Add9/2
  Gain1/1 -> Subtract/2
  vyl/1 -> Dot Product/1, Subtract4/1, Subtract3/1, Add10/1, Add9/1
  Add9/1 -> vy1/1
  Gain2/1 -> Add6/1
  Add4/1 -> Gain3/1
  Subtract4/1 -> vy4/1
  Subtract1/1 -> vx1/1
  Add6/1 -> Gain8/1
  Add10/1 -> vy2/1
  Dot Product/1 -> Add2/1
  Gain7/1 -> Subtract4/2, Subtract3/2
  Gain5/1 -> Add8/2, Subtract2/2, Add7/2, Subtract1/2
  Subtract2/1 -> vx3/1
  Subtract/1 -> Display1/1, vyld/1
  Dot Product1/1 -> Subtract/1
  Add7/1 -> vx2/1
  Add5/1 -> Gain4/1
  Gain3/1 -> Add6/2
  Add2/1 -> Display/1, To Workspace/1, vxld/1
  Gain/1 -> Add2/2
  fy4/1 -> Add5/2, Add1/4
  fy2/1 -> Add4/2, Add1/2
  fy3/1 -> Add5/1, Add1/3
  fy1/1 -> Add1/1, Add4/1
  fx4/1 -> Add3/4, Add/4
  fx2/1 -> Add3/2, Add/2
  fx3/1 -> Add3/3, Add/3
  fx1/1 -> Add3/1, Add/1
  Gain4/1 -> Add6/3
  Gain8/1 -> Display2/1, yawd/1

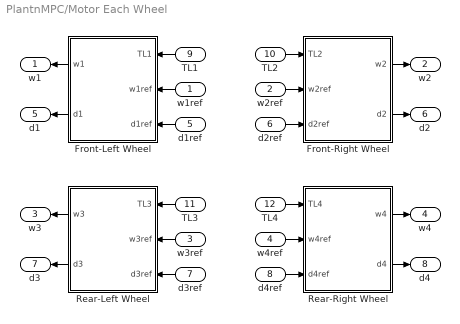
== system PlantnMPC/Motor Each Wheel ==
  w1ref : Inport
  w2ref : Inport  Port=2
  w3ref : Inport  Port=3
  w4ref : Inport  Port=4
  d1ref : Inport  Port=5
  d2ref : Inport  Port=6
  d3ref : Inport  Port=7
  d4ref : Inport  Port=8
  TL1 : Inport  Port=9
  TL2 : Inport  Port=10
  TL3 : Inport  Port=11
  TL4 : Inport  Port=12
  Front-Left Wheel : Subsystem
  Front-Right Wheel : Subsystem
  Rear-Left Wheel : Subsystem
  Rear-Right Wheel : Subsystem
  w1 : Outport
  w2 : Outport  Port=2
  w3 : Outport  Port=3
  w4 : Outport  Port=4
  d1 : Outport  Port=5
  d2 : Outport  Port=6
  d3 : Outport  Port=7
  d4 : Outport  Port=8
  wires:
  TL1/1 -> Front-Left Wheel/1(TL1)
  w1ref/1 -> Front-Left Wheel/2(w1ref)
  w2ref/1 -> Front-Right Wheel/2(w2ref)
  Front-Left Wheel/1(w1) -> w1/1
  Front-Right Wheel/1(w2) -> w2/1
  d1ref/1 -> Front-Left Wheel/3(d1ref)
  w4ref/1 -> Rear-Right Wheel/2(w4ref)
  d2ref/1 -> Front-Right Wheel/3(d2ref)
  Front-Right Wheel/2(d2) -> d2/1
  Front-Left Wheel/2(d1) -> d1/1
  Rear-Right Wheel/1(w4) -> w4/1
  Rear-Left Wheel/1(w3) -> w3/1
  w3ref/1 -> Rear-Left Wheel/2(w3ref)
  d3ref/1 -> Rear-Left Wheel/3(d3ref)
  TL2/1 -> Front-Right Wheel/1(TL2)
  TL3/1 -> Rear-Left Wheel/1(TL3)
  Rear-Left Wheel/2(d3) -> d3/1
  d4ref/1 -> Rear-Right Wheel/3(d4ref)
  TL4/1 -> Rear-Right Wheel/1(TL4)
  Rear-Right Wheel/2(d4) -> d4/1

== system PlantnMPC/NMPC_N//GMRES ==
  States : Inport
  Dynamic TVP : Inport  Port=2
  Frozen TVP : Inport  Port=3
  Solver : MATLAB Function  TreatAsAtomicUnit=on
  U0 : UnitDelay  InitialCondition=U0  SampleTime=-1  HasFrameUpgradeWarning=on
  dU0 : UnitDelay  InitialCondition=dU0  SampleTime=-1  HasFrameUpgradeWarning=on
  Controls : Outport
  wires:
  Dynamic TVP/1 -> Solver/4(TVP)
  dU0/1 -> Solver/1(dU0)
  Solver/1(dU) -> dU0/1
  U0/1 -> Solver/2(U0)
  Solver/2(U) -> U0/1
  Solver/3(Control) -> Controls/1
  Frozen TVP/1 -> Solver/5(TVP_f)
  States/1 -> Solver/3(x0)

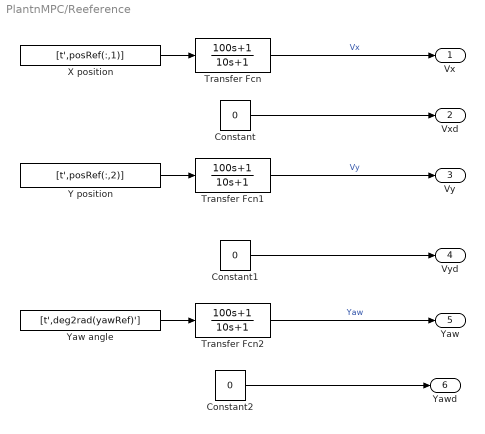
== system PlantnMPC/Reeference ==
  Constant : Constant  Value=0
  Constant1 : Constant  Value=0
  Constant2 : Constant  Value=0
  Transfer Fcn : TransferFcn  Numerator=[100 1]  Denominator=[10 1]
  Transfer Fcn1 : TransferFcn  Numerator=[100 1]  Denominator=[10 1]
  Transfer Fcn2 : TransferFcn  Numerator=[100 1]  Denominator=[10 1]
  X position : FromWorkspace  VariableName=[t',posRef(:,1)]
  Y position : FromWorkspace  VariableName=[t',posRef(:,2)]
  Yaw angle : FromWorkspace  VariableName=[t',deg2rad(yawRef)']
  Vx : Outport
  Vxd : Outport  Port=2
  Vy : Outport  Port=3
  Vyd : Outport  Port=4
  Yaw : Outport  Port=5
  Yawd : Outport  Port=6
  wires:
  X position/1 -> Transfer Fcn/1
  Yaw angle/1 -> Transfer Fcn2/1
  Y position/1 -> Transfer Fcn1/1
  Transfer Fcn1/1 -> Vy/1  "Vy"
  Transfer Fcn/1 -> Vx/1  "Vx"
  Transfer Fcn2/1 -> Yaw/1  "Yaw"
  Constant/1 -> Vxd/1
  Constant1/1 -> Vyd/1
  Constant2/1 -> Yawd/1

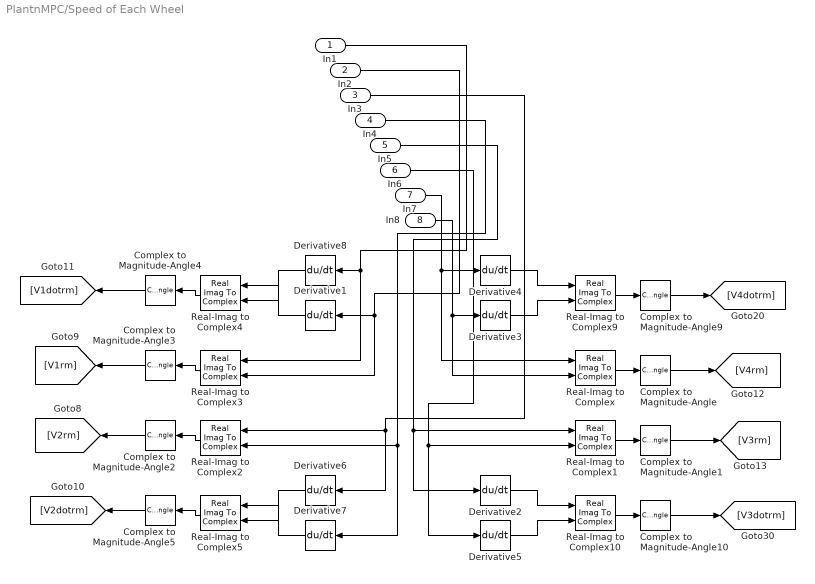
== system PlantnMPC/Speed of Each Wheel ==
  In1 : Inport
  In2 : Inport  Port=2
  In3 : Inport  Port=3
  In4 : Inport  Port=4
  In5 : Inport  Port=5
  In6 : Inport  Port=6
  In7 : Inport  Port=7
  In8 : Inport  Port=8
  Complex to Magnitude-Angle{,1..5,9..10} (8 alike) : ComplexToMagnitudeAngle  Output=Magnitude
  Derivative{1..8} (8 alike) : Derivative
  Real-Imag to Complex{,1..5,9..10} (8 alike) : RealImagToComplex
  wires:
  In2/1 -> Real-Imag to Complex3/2, Derivative1/1
  Complex to Magnitude-Angle2/1 -> [V2rm]
  In8/1 -> Real-Imag to Complex/2, Derivative3/1
  Real-Imag to Complex9/1 -> Complex to Magnitude-Angle9/1
  Real-Imag to Complex/1 -> Complex to Magnitude-Angle/1
  In3/1 -> Derivative6/1, Real-Imag to Complex2/1
  Complex to Magnitude-Angle5/1 -> [V2dotrm]
  In1/1 -> Real-Imag to Complex3/1, Derivative8/1
  Derivative7/1 -> Real-Imag to Complex5/1
  Real-Imag to Complex1/1 -> Complex to Magnitude-Angle1/1
  Real-Imag to Complex3/1 -> Complex to Magnitude-Angle3/1
  Complex to Magnitude-Angle1/1 -> [V3rm]
  In4/1 -> Derivative7/1, Real-Imag to Complex2/2
  Complex to Magnitude-Angle4/1 -> [V1dotrm]
  In6/1 -> Derivative5/1, Real-Imag to Complex1/2
  Complex to Magnitude-Angle3/1 -> [V1rm]
  Derivative8/1 -> Real-Imag to Complex4/2
  Real-Imag to Complex10/1 -> Complex to Magnitude-Angle10/1
  Derivative2/1 -> Real-Imag to Complex10/1
  Complex to Magnitude-Angle10/1 -> [V3dotrm]
  In7/1 -> Real-Imag to Complex/1, Derivative4/1
  Derivative3/1 -> Real-Imag to Complex9/2
  Complex to Magnitude-Angle9/1 -> [V4dotrm]
  In5/1 -> Derivative2/1, Real-Imag to Complex1/1
  Complex to Magnitude-Angle/1 -> [V4rm]
  Derivative4/1 -> Real-Imag to Complex9/1
  Derivative5/1 -> Real-Imag to Complex10/2
  Real-Imag to Complex5/1 -> Complex to Magnitude-Angle5/1
  Real-Imag to Complex2/1 -> Complex to Magnitude-Angle2/1
  Derivative1/1 -> Real-Imag to Complex4/1
  Derivative6/1 -> Real-Imag to Complex5/2
  Real-Imag to Complex4/1 -> Complex to Magnitude-Angle4/1

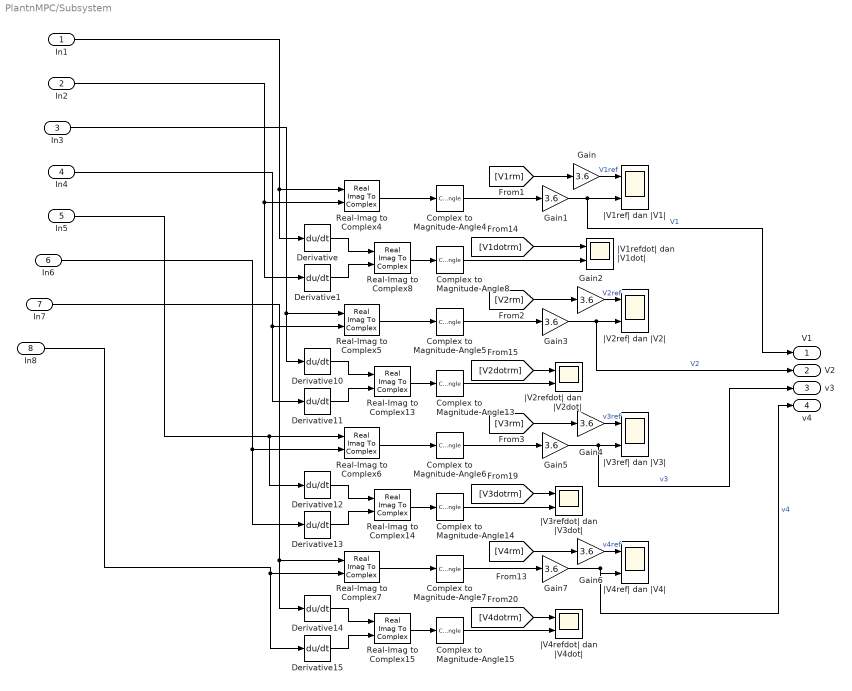
== system PlantnMPC/Subsystem ==
  In1 : Inport
  In2 : Inport  Port=2
  In3 : Inport  Port=3
  In4 : Inport  Port=4
  In5 : Inport  Port=5
  In6 : Inport  Port=6
  In7 : Inport  Port=7
  In8 : Inport  Port=8
  Complex to Magnitude-Angle{4..8,13..15} (8 alike) : ComplexToMagnitudeAngle  Output=Magnitude
  Derivative{,1,10..15} (8 alike) : Derivative
  Gain{,1..7} (8 alike) : Gain  Gain=3.6
  Real-Imag to Complex{4..8,13..15} (8 alike) : RealImagToComplex
  |V1refdot| dan |V1dot| : Scope  NumInputPorts=2
  |V1ref| dan |V1| : Scope  NumInputPorts=2
  |V2refdot| dan |V2dot| : Scope  NumInputPorts=2
  |V2ref| dan |V2| : Scope  NumInputPorts=2
  |V3refdot| dan |V3dot| : Scope  NumInputPorts=2
  |V3ref| dan |V3| : Scope  NumInputPorts=2
  |V4refdot| dan |V4dot| : Scope  NumInputPorts=2
  |V4ref| dan |V4| : Scope  NumInputPorts=2
  V1 : Outport
  V2 : Outport  Port=2
  v3 : Outport  Port=3
  v4 : Outport  Port=4
  wires:
  Real-Imag to Complex7/1 -> Complex to Magnitude-Angle7/1
  In8/1 -> Derivative15/1, Real-Imag to Complex7/2
  Derivative13/1 -> Real-Imag to Complex14/2
  In6/1 -> Derivative13/1, Real-Imag to Complex6/2
  Real-Imag to Complex15/1 -> Complex to Magnitude-Angle15/1
  Real-Imag to Complex13/1 -> Complex to Magnitude-Angle13/1
  Gain3/1 -> V2/1, |V2ref| dan |V2|/2  "V2"
  Gain2/1 -> |V2ref| dan |V2|/1  "V2ref"
  Derivative1/1 -> Real-Imag to Complex8/2
  Complex to Magnitude-Angle6/1 -> Gain5/1
  In1/1 -> Derivative/1, Real-Imag to Complex4/1
  Gain5/1 -> v3/1, |V3ref| dan |V3|/2  "v3"
  Gain7/1 -> v4/1, |V4ref| dan |V4|/2  "v4"
  In4/1 -> Derivative11/1, Real-Imag to Complex5/2
  [V4dotrm] -> |V4refdot| dan |V4dot|/1
  [V1rm] -> Gain/1
  Derivative14/1 -> Real-Imag to Complex15/1
  Derivative10/1 -> Real-Imag to Complex13/1
  Derivative12/1 -> Real-Imag to Complex14/1
  Real-Imag to Complex8/1 -> Complex to Magnitude-Angle8/1
  In5/1 -> Derivative12/1, Real-Imag to Complex6/1
  Real-Imag to Complex4/1 -> Complex to Magnitude-Angle4/1
  Gain/1 -> |V1ref| dan |V1|/1  "V1ref"
  Complex to Magnitude-Angle13/1 -> |V2refdot| dan |V2dot|/2
  Real-Imag to Complex14/1 -> Complex to Magnitude-Angle14/1
  Complex to Magnitude-Angle7/1 -> Gain7/1
  Complex to Magnitude-Angle5/1 -> Gain3/1
  Derivative/1 -> Real-Imag to Complex8/1
  [V4rm] -> Gain6/1
  [V2dotrm] -> |V2refdot| dan |V2dot|/1
  Complex to Magnitude-Angle15/1 -> |V4refdot| dan |V4dot|/2
  In2/1 -> Derivative1/1, Real-Imag to Complex4/2
  Complex to Magnitude-Angle4/1 -> Gain1/1
  [V3dotrm] -> |V3refdot| dan |V3dot|/1
  [V1dotrm] -> |V1refdot| dan |V1dot|/1
  Gain1/1 -> |V1ref| dan |V1|/2, V1/1  "V1"
  Real-Imag to Complex6/1 -> Complex to Magnitude-Angle6/1
  Real-Imag to Complex5/1 -> Complex to Magnitude-Angle5/1
  Complex to Magnitude-Angle8/1 -> |V1refdot| dan |V1dot|/2
  [V3rm] -> Gain4/1
  [V2rm] -> Gain2/1
  Gain6/1 -> |V4ref| dan |V4|/1  "v4ref"
  Gain4/1 -> |V3ref| dan |V3|/1  "v3ref"
  Derivative11/1 -> Real-Imag to Complex13/2
  Complex to Magnitude-Angle14/1 -> |V3refdot| dan |V3dot|/2
  Derivative15/1 -> Real-Imag to Complex15/2
  In3/1 -> Derivative10/1, Real-Imag to Complex5/1
  In7/1 -> Derivative14/1, Real-Imag to Complex7/1

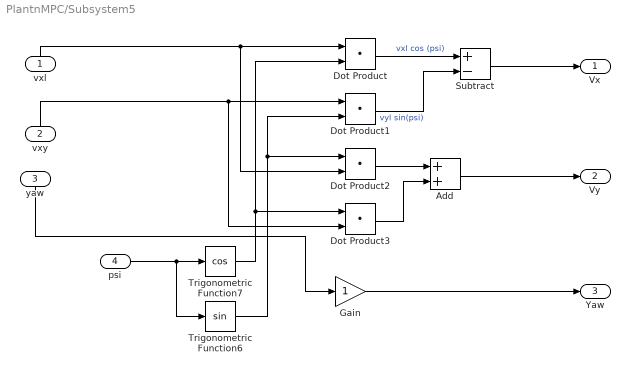
== system PlantnMPC/Subsystem5 ==
  vxl : Inport
  vxy : Inport  Port=2
  yaw : Inport  Port=3
  psi : Inport  Port=4
  Add : Sum
  Dot Product{,1..3} (4 alike) : DotProduct  InputSameDT=on  OutDataTypeStr=Inherit: Inherit via internal rule
  Gain : Gain
  Subtract : Sum  Inputs=+-
  Trigonometric Function6 : Trigonometry
  Trigonometric Function7 : Trigonometry  Operator=cos
  Vx : Outport
  Vy : Outport  Port=2
  Yaw : Outport  Port=3
  wires:
  Gain/1 -> Yaw/1
  Dot Product1/1 -> Subtract/2  "vyl sin(psi)"
  Subtract/1 -> Vx/1
  Dot Product2/1 -> Add/1
  yaw/1 -> Gain/1
  vxl/1 -> Dot Product2/2, Dot Product/1
  vxy/1 -> Dot Product3/2, Dot Product1/1
  Dot Product3/1 -> Add/2
  psi/1 -> Trigonometric Function6/1, Trigonometric Function7/1
  Trigonometric Function7/1 -> Dot Product3/1, Dot Product/2
  Trigonometric Function6/1 -> Dot Product2/1, Dot Product1/2
  Add/1 -> Vy/1
  Dot Product/1 -> Subtract/1  "vxl cos (psi)"

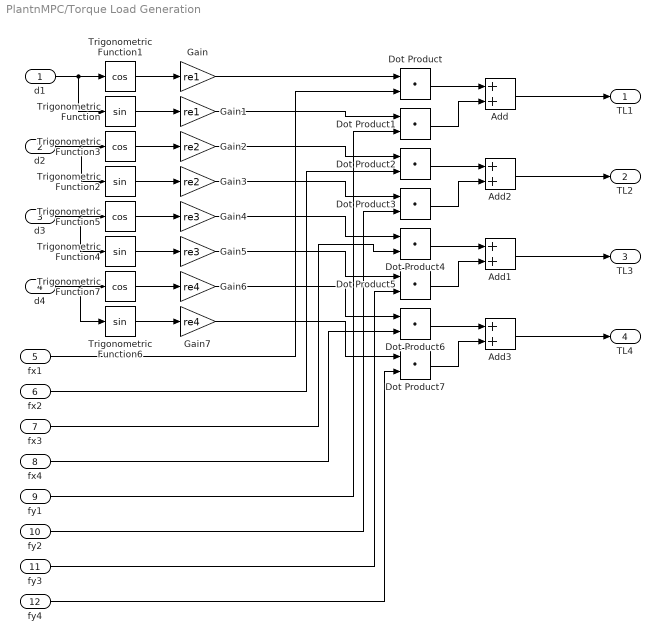
== system PlantnMPC/Torque Load Generation ==
  d1 : Inport
  d2 : Inport  Port=2
  d3 : Inport  Port=3
  d4 : Inport  Port=4
  fx1 : Inport  Port=5
  fx2 : Inport  Port=6
  fx3 : Inport  Port=7
  fx4 : Inport  Port=8
  fy1 : Inport  Port=9
  fy2 : Inport  Port=10
  fy3 : Inport  Port=11
  fy4 : Inport  Port=12
  Add{,1..3} (4 alike) : Sum
  Dot Product{,1..7} (8 alike) : DotProduct  InputSameDT=on  OutDataTypeStr=Inherit: Inherit via internal rule
  Gain : Gain  Gain=re1
  Gain1 : Gain  Gain=re1
  Gain2 : Gain  Gain=re2
  Gain3 : Gain  Gain=re2
  Gain4 : Gain  Gain=re3
  Gain5 : Gain  Gain=re3
  Gain6 : Gain  Gain=re4
  Gain7 : Gain  Gain=re4
  Trigonometric Function{,2,4,6} (4 alike) : Trigonometry
  Trigonometric Function{1,3,5,7} (4 alike) : Trigonometry  Operator=cos
  TL1 : Outport
  TL2 : Outport  Port=2
  TL3 : Outport  Port=3
  TL4 : Outport  Port=4
  wires:
  Gain3/1 -> Dot Product3/1
  fy2/1 -> Dot Product3/2
  Dot Product2/1 -> Add2/1
  fx2/1 -> Dot Product2/2
  Add1/1 -> TL3/1
  Gain2/1 -> Dot Product2/1
  fx1/1 -> Dot Product/2
  d3/1 -> Trigonometric Function4/1, Trigonometric Function5/1
  Trigonometric Function4/1 -> Gain5/1
  Dot Product1/1 -> Add/2
  fy1/1 -> Dot Product1/2
  Dot Product5/1 -> Add1/2
  Dot Product7/1 -> Add3/2
  Add2/1 -> TL2/1
  Dot Product/1 -> Add/1
  Gain6/1 -> Dot Product6/1
  Gain5/1 -> Dot Product5/1
  d2/1 -> Trigonometric Function2/1, Trigonometric Function3/1
  Gain1/1 -> Dot Product1/1
  fx4/1 -> Dot Product6/2
  d1/1 -> Trigonometric Function/1, Trigonometric Function1/1
  fy4/1 -> Dot Product7/2
  Dot Product3/1 -> Add2/2
  Trigonometric Function2/1 -> Gain3/1
  Trigonometric Function6/1 -> Gain7/1
  Dot Product6/1 -> Add3/1
  Trigonometric Function1/1 -> Gain/1
  Add/1 -> TL1/1
  Add3/1 -> TL4/1
  fx3/1 -> Dot Product4/2
  Trigonometric Function7/1 -> Gain6/1
  Trigonometric Function3/1 -> Gain2/1
  Trigonometric Function/1 -> Gain1/1
  Gain4/1 -> Dot Product4/1
  d4/1 -> Trigonometric Function6/1, Trigonometric Function7/1
  Gain/1 -> Dot Product/1
  Trigonometric Function5/1 -> Gain4/1
  Gain7/1 -> Dot Product7/1
  Dot Product4/1 -> Add1/1
  fy3/1 -> Dot Product5/2

== system PlantnMPC/Motor Each Wheel/Front-Left Wheel ==
  TL1 : Inport
  w1ref : Inport  Port=2
  d1ref : Inport  Port=3
  Driving Motor 1 : Subsystem  mask(MCS){}
      mask help: Kontroller X
  Steering Motor 1 : Subsystem  mask(MCS){}
      mask help: Kontroller X
  w1 : Outport
  d1 : Outport  Port=2
  wires:
  Steering Motor 1/1(d1) -> d1/1
  TL1/1 -> Driving Motor 1/1(TL1)
  d1ref/1 -> Steering Motor 1/1(d1ref)
  Driving Motor 1/1(w1) -> w1/1
  w1ref/1 -> Driving Motor 1/2(w1ref)

== system PlantnMPC/Motor Each Wheel/Front-Right Wheel ==
  TL2 : Inport
  w2ref : Inport  Port=2
  d2ref : Inport  Port=3
  Driving Motor 2 : Subsystem  mask(MCS){}
      mask help: Kontroller X
  Steering Motor 2 : Subsystem  mask(MCS){}
      mask help: Kontroller X
  w2 : Outport
  d2 : Outport  Port=2
  wires:
  Steering Motor 2/1(d2) -> d2/1
  TL2/1 -> Driving Motor 2/1(TL2)
  d2ref/1 -> Steering Motor 2/1(d2ref)
  Driving Motor 2/1(w2) -> w2/1
  w2ref/1 -> Driving Motor 2/2(w2ref)

== system PlantnMPC/Motor Each Wheel/Rear-Left Wheel ==
  TL3 : Inport
  w3ref : Inport  Port=2
  d3ref : Inport  Port=3
  Driving Motor 3 : Subsystem  mask(MCS){}
      mask help: Kontroller X
  Steering Motor 3 : Subsystem  mask(MCS){}
      mask help: Kontroller X
  w3 : Outport
  d3 : Outport  Port=2
  wires:
  Steering Motor 3/1(d3) -> d3/1
  TL3/1 -> Driving Motor 3/1(TL3)
  d3ref/1 -> Steering Motor 3/1(d3ref)
  Driving Motor 3/1(w3) -> w3/1
  w3ref/1 -> Driving Motor 3/2(w3ref)

== system PlantnMPC/Motor Each Wheel/Rear-Right Wheel ==
  TL4 : Inport
  w4ref : Inport  Port=2
  d4ref : Inport  Port=3
  Driving Motor 4 : Subsystem  mask(MCS){}
      mask help: Kontroller X
  Steering Motor 4 : Subsystem  mask(MCS){}
      mask help: Kontroller X
  w4 : Outport
  d4 : Outport  Port=2
  wires:
  Steering Motor 4/1(d4) -> d4/1
  TL4/1 -> Driving Motor 4/1(TL4)
  d4ref/1 -> Steering Motor 4/1(d4ref)
  Driving Motor 4/1(w4) -> w4/1
  w4ref/1 -> Driving Motor 4/2(w4ref)

== system PlantnMPC/Motor Each Wheel/Front-Left Wheel/Driving Motor 1 ==
  TL1 : Inport
  w1ref : Inport  Port=2
  Display1 : Display
  Gain8 : Gain  Gain=2
  Gain9 : Gain  Gain=2
  Speed Controller : TransferFcn  Numerator=[30 60]  Denominator=[1 0]
  Sum21 : Sum  Inputs=|+-
  Sum22 : Sum  Inputs=|++
  Sum23 : Sum  Inputs=-+|
  Sum24 : Sum  Inputs=+-
  Terminator : Terminator
  Transfer Fcn21 : TransferFcn  Denominator=[0.36 0.57]
  Transfer Fcn22 : TransferFcn  Numerator=[0.36 0.57]  Denominator=[0.002 2]
  noise filter : TransferFcn  Denominator=[0.001 1]
  w1 : Outport
  wires:
  Sum22/1 -> noise filter/1, Gain8/1  "error 2"
  Gain8/1 -> Sum23/2
  Transfer Fcn22/1 -> Sum24/2
  Speed Controller/1 -> Sum22/1
  noise filter/1 -> Sum24/1
  Sum24/1 -> Sum22/2, Gain9/1
  Sum21/1 -> Speed Controller/1  "error 1"
  Sum23/1 -> Transfer Fcn21/1
  Transfer Fcn21/1 -> w1/1, Sum21/2, Transfer Fcn22/1  "out"
  TL1/1 -> Display1/1, Sum23/1
  w1ref/1 -> Sum21/1
  Gain9/1 -> Terminator/1

== system PlantnMPC/Motor Each Wheel/Front-Left Wheel/Steering Motor 1 ==
  d1ref : Inport
  Sum21 : Sum  Inputs=|+-
  Transfer Fcn : TransferFcn  Numerator=[100]  Denominator=[10 1]
  d1 : Outport
  wires:
  d1ref/1 -> Sum21/1
  Sum21/1 -> Transfer Fcn/1  "error 1"
  Transfer Fcn/1 -> Sum21/2, d1/1

== system PlantnMPC/Motor Each Wheel/Front-Right Wheel/Driving Motor 2 ==
  TL2 : Inport
  w2ref : Inport  Port=2
  Display1 : Display
  Gain8 : Gain  Gain=2
  Gain9 : Gain  Gain=2
  Speed Controller : TransferFcn  Numerator=[30 60]  Denominator=[1 0]
  Sum21 : Sum  Inputs=|+-
  Sum22 : Sum  Inputs=|++
  Sum23 : Sum  Inputs=-+|
  Sum24 : Sum  Inputs=+-
  Terminator : Terminator
  Transfer Fcn21 : TransferFcn  Denominator=[0.36 0.57]
  Transfer Fcn22 : TransferFcn  Numerator=[0.36 0.57]  Denominator=[0.002 2]
  noise filter : TransferFcn  Denominator=[0.001 1]
  w2 : Outport
  wires:
  Sum22/1 -> noise filter/1, Gain8/1  "error 2"
  Gain8/1 -> Sum23/2
  Transfer Fcn22/1 -> Sum24/2
  Speed Controller/1 -> Sum22/1
  noise filter/1 -> Sum24/1
  Sum24/1 -> Sum22/2, Gain9/1
  Sum21/1 -> Speed Controller/1  "error 1"
  Sum23/1 -> Transfer Fcn21/1
  Transfer Fcn21/1 -> w2/1, Sum21/2, Transfer Fcn22/1  "out"
  TL2/1 -> Display1/1, Sum23/1
  w2ref/1 -> Sum21/1
  Gain9/1 -> Terminator/1

== system PlantnMPC/Motor Each Wheel/Front-Right Wheel/Steering Motor 2 ==
  d2ref : Inport
  Sum21 : Sum  Inputs=|+-
  Transfer Fcn : TransferFcn  Numerator=[100]  Denominator=[10 1]
  d2 : Outport
  wires:
  d2ref/1 -> Sum21/1
  Sum21/1 -> Transfer Fcn/1  "error 1"
  Transfer Fcn/1 -> Sum21/2, d2/1

== system PlantnMPC/Motor Each Wheel/Rear-Left Wheel/Driving Motor 3 ==
  TL3 : Inport
  w3ref : Inport  Port=2
  Display1 : Display
  Gain8 : Gain  Gain=2
  Gain9 : Gain  Gain=2
  Speed Controller : TransferFcn  Numerator=[30 60]  Denominator=[1 0]
  Sum21 : Sum  Inputs=|+-
  Sum22 : Sum  Inputs=|++
  Sum23 : Sum  Inputs=-+|
  Sum24 : Sum  Inputs=+-
  Terminator : Terminator
  Transfer Fcn21 : TransferFcn  Denominator=[0.36 0.57]
  Transfer Fcn22 : TransferFcn  Numerator=[0.36 0.57]  Denominator=[0.002 2]
  noise filter : TransferFcn  Denominator=[0.001 1]
  w3 : Outport
  wires:
  Sum22/1 -> noise filter/1, Gain8/1  "error 2"
  Gain8/1 -> Sum23/2
  Transfer Fcn22/1 -> Sum24/2
  Speed Controller/1 -> Sum22/1
  noise filter/1 -> Sum24/1
  Sum24/1 -> Sum22/2, Gain9/1
  Sum21/1 -> Speed Controller/1  "error 1"
  Sum23/1 -> Transfer Fcn21/1
  Transfer Fcn21/1 -> w3/1, Sum21/2, Transfer Fcn22/1  "out"
  TL3/1 -> Display1/1, Sum23/1
  w3ref/1 -> Sum21/1
  Gain9/1 -> Terminator/1

== system PlantnMPC/Motor Each Wheel/Rear-Left Wheel/Steering Motor 3 ==
  d3ref : Inport
  Sum21 : Sum  Inputs=|+-
  Transfer Fcn : TransferFcn  Numerator=[100]  Denominator=[10 1]
  d3 : Outport
  wires:
  d3ref/1 -> Sum21/1
  Transfer Fcn/1 -> Sum21/2, d3/1
  Sum21/1 -> Transfer Fcn/1  "error 1"

== system PlantnMPC/Motor Each Wheel/Rear-Right Wheel/Driving Motor 4 ==
  TL4 : Inport
  w4ref : Inport  Port=2
  Display1 : Display
  Gain8 : Gain  Gain=2
  Gain9 : Gain  Gain=2
  Speed Controller : TransferFcn  Numerator=[30 60]  Denominator=[1 0]
  Sum21 : Sum  Inputs=|+-
  Sum22 : Sum  Inputs=|++
  Sum23 : Sum  Inputs=-+|
  Sum24 : Sum  Inputs=+-
  Terminator : Terminator
  Transfer Fcn21 : TransferFcn  Denominator=[0.36 0.57]
  Transfer Fcn22 : TransferFcn  Numerator=[0.36 0.57]  Denominator=[0.002 2]
  noise filter : TransferFcn  Denominator=[0.001 1]
  w4 : Outport
  wires:
  Sum22/1 -> noise filter/1, Gain8/1  "error 2"
  Gain8/1 -> Sum23/2
  Transfer Fcn22/1 -> Sum24/2
  Speed Controller/1 -> Sum22/1
  noise filter/1 -> Sum24/1
  Sum24/1 -> Sum22/2, Gain9/1
  Sum21/1 -> Speed Controller/1  "error 1"
  Sum23/1 -> Transfer Fcn21/1
  Transfer Fcn21/1 -> w4/1, Sum21/2, Transfer Fcn22/1  "out"
  TL4/1 -> Display1/1, Sum23/1
  w4ref/1 -> Sum21/1
  Gain9/1 -> Terminator/1

== system PlantnMPC/Motor Each Wheel/Rear-Right Wheel/Steering Motor 4 ==
  d4ref : Inport
  Sum21 : Sum  Inputs=|+-
  Transfer Fcn : TransferFcn  Numerator=[100]  Denominator=[10 1]
  d4 : Outport
  wires:
  d4ref/1 -> Sum21/1
  Sum21/1 -> Transfer Fcn/1  "error 1"
  Transfer Fcn/1 -> Sum21/2, d4/1

== matlab function PlantnMPC/PlantNMPC ==
  data: x input; u input; xdot output
function xdot = UEV(x,u)
Xk1=x(1);
Xk2=x(2);
Xk3=x(3);
Xk4=x(4);
Xk5=x(5);
Xk6=x(6);
Uk1=u(1);
Uk2=u(2);
Uk3=u(3);
Uk4=u(4);
Uk5=u(5);
Uk6=u(6);
Uk7=u(7);
Uk8=u(8);
xdot=zeros(6,1);
xdot(1)=Xk1;
xdot(2)=((Uk1+Uk2+Uk3+Uk4)/1960)+(Xk2*Xk3);
xdot(3)=Xk3;
xdot(4)=((Uk5+Uk6+Uk7+Uk8)/1960)-(Xk1*Xk2);
xdot(5)=Xk5;
xdot(6)=((1.22*(Uk5+Uk6))-(1.36*(Uk7+Uk8))+(0.75*(Uk2+Uk4))-(0.75*(Uk1+Uk3)))/1536.7;

== matlab function PlantnMPC/EVloop1&2(3)-(6)1/MATLAB Function1 ==
  data: Nx input; Ny input; m input; g input; h input; ld input; lf input; lr input; kro input; kfo input; fz1 output; fz2 output; fz3 output; fz4 output
function [fz1,fz2,fz3,fz4]  = invers(Nx,Ny,m,g,h,ld,lf,lr,kro,kfo)

N=[Nx Ny]';
Fzs=(m*g/2)*[lr/(lf+lr) lr/(lf+lr) lf/(lf+lr) lf/(lf+lr)]';
G=(h/(2*ld))*[ld/(lf+lr) ld/(lf+lr) -ld/(lf+lr) -ld/(lf+lr);
    kfo/(kfo+kro) -kfo/(kfo+kro) kro/(kfo+kro) -kro/(kfo+kro)]';
miu=eye(4,4)+(G*N);
fz=miu\Fzs;
fz1=fz(1,1);
fz2=fz(2,1);
fz3=fz(3,1);
fz4=fz(4,1);

== matlab function PlantnMPC/NMPC_N//GMRES/Solver ==
  data: dU0 input; dU output; U0 input; x0 input; TVP input; U output; Control output; TVP_f input
%% NGMRES  NGMRES NGMRES
function [dU,U,Control] = NMPCBlock(dU0,U0,x0,TVP,TVP_f)
[dU,U,Control]=NMPC(dU0,U0,x0,TVP,TVP_f);
